simulink model "tricopter_simulation"  (Simulink 7.8)
settings: Solver=FixedStepDiscrete  StartTime=0.0  StopTime=10  FixedStep=dt_sim  RelTol=1e-3
InitFcn:
  | Init
values from neighbouring files (symbols this model uses):
  act_latency = 1*dt_sim    (= 0.005)    [Init.m]
  D = 1    [Init.m]
  dt_sim = 0.005    [Init.m]
  gvec = [0 0 9.81]'    [Init.m]
  J = diag([0.25*m*(D/2)^2 0.25*m*(D/2)^2 0.5*m*(D/2)^2])    [Init.m]
  k = 0.0000192    (= 1.92e-05)    [Init.m]
  L = 0.5    [Init.m]
  m = 1    [Init.m]
  max_rpm = 7000*pi/30    (= 733.038285838)    [Init.m]
  min_rpm = 0    [Init.m]
  rho = 1.26    [Init.m]
undefined symbols (not defined in the file or in its folder): DiscIntNeverNeededParam, waitfortreal
libraries: animation_lib x1, simulink x1
(part 2 of 2)

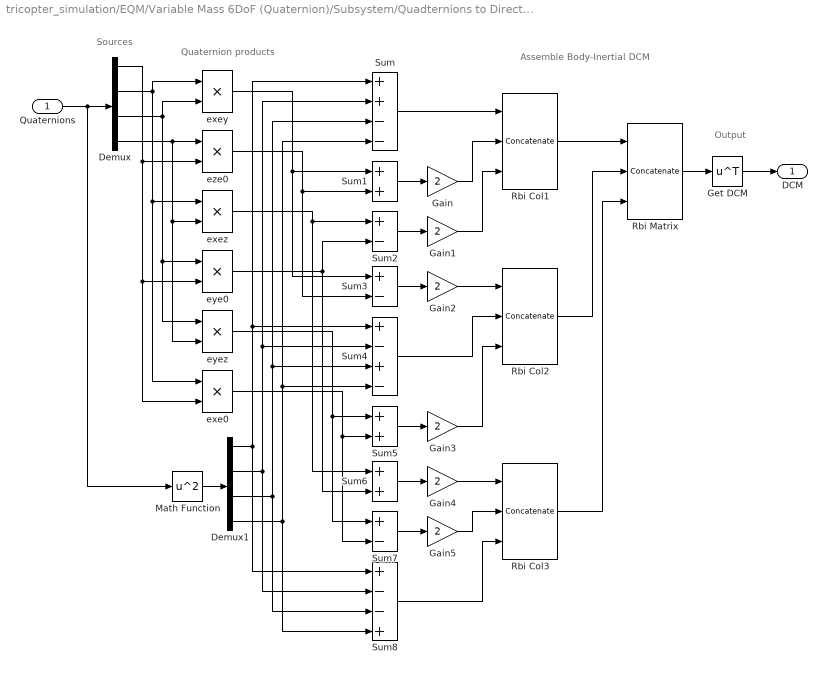
== system tricopter_simulation/EQM/Variable Mass 6DoF (Quaternion)/Subsystem/Quadternions to Direct Cosine Matrix ==
  note: Output
  note: Quaternion products
  note: Assemble Body-Inertial DCM
  note: Sources
  Quaternions : Inport  PortDimensions=[4 1]
  Demux : Demux
  Demux1 : Demux
  Gain{,1..5} (6 alike) : Gain  Gain=2  SaturateOnIntegerOverflow=on  OutDataTypeStr=Inherit: Same as input  ParamDataTypeStr=Inherit: Same as input
  Get DCM : Math  Operator=transpose  SaturateOnIntegerOverflow=on
  Math Function : Math  Operator=square  SaturateOnIntegerOverflow=on
  Rbi Matrix : Concatenate  NumInputs=3  Mode=Multidimensional array  ConcatenateDimension=2
  Rbi Col1 : Concatenate  NumInputs=3  Mode=Multidimensional array
  Rbi Col2 : Concatenate  NumInputs=3  Mode=Multidimensional array
  Rbi Col3 : Concatenate  NumInputs=3  Mode=Multidimensional array
  Sum : Sum  Inputs=++--  SaturateOnIntegerOverflow=on  InputSameDT=on  OutDataTypeStr=Inherit: Same as first input
  Sum1 : Sum  SaturateOnIntegerOverflow=on  InputSameDT=on  OutDataTypeStr=Inherit: Same as first input
  Sum2 : Sum  Inputs=+-  SaturateOnIntegerOverflow=on  InputSameDT=on  OutDataTypeStr=Inherit: Same as first input
  Sum3 : Sum  Inputs=+-  SaturateOnIntegerOverflow=on  InputSameDT=on  OutDataTypeStr=Inherit: Same as first input
  Sum4 : Sum  Inputs=+-+-  SaturateOnIntegerOverflow=on  InputSameDT=on  OutDataTypeStr=Inherit: Same as first input
  Sum5 : Sum  SaturateOnIntegerOverflow=on  InputSameDT=on  OutDataTypeStr=Inherit: Same as first input
  Sum6 : Sum  SaturateOnIntegerOverflow=on  InputSameDT=on  OutDataTypeStr=Inherit: Same as first input
  Sum7 : Sum  Inputs=+-  SaturateOnIntegerOverflow=on  InputSameDT=on  OutDataTypeStr=Inherit: Same as first input
  Sum8 : Sum  Inputs=+--+  SaturateOnIntegerOverflow=on  InputSameDT=on  OutDataTypeStr=Inherit: Same as first input
  exe0 : Product  SaturateOnIntegerOverflow=on  InputSameDT=on  OutDataTypeStr=Inherit: Same as first input
  exey : Product  SaturateOnIntegerOverflow=on  InputSameDT=on  OutDataTypeStr=Inherit: Same as first input
  exez : Product  SaturateOnIntegerOverflow=on  InputSameDT=on  OutDataTypeStr=Inherit: Same as first input
  eye0 : Product  SaturateOnIntegerOverflow=on  InputSameDT=on  OutDataTypeStr=Inherit: Same as first input
  eyez : Product  SaturateOnIntegerOverflow=on  InputSameDT=on  OutDataTypeStr=Inherit: Same as first input
  eze0 : Product  SaturateOnIntegerOverflow=on  InputSameDT=on  OutDataTypeStr=Inherit: Same as first input
  DCM : Outport
  wires:
  Get DCM/1 -> DCM/1
  Rbi Matrix/1 -> Get DCM/1
  Sum8/1 -> Rbi Col3/3
  Gain5/1 -> Rbi Col3/2
  Gain4/1 -> Rbi Col3/1
  Rbi Col3/1 -> Rbi Matrix/3
  Sum7/1 -> Gain5/1
  Sum6/1 -> Gain4/1
  Rbi Col2/1 -> Rbi Matrix/2
  Gain3/1 -> Rbi Col2/3
  Sum4/1 -> Rbi Col2/2
  Gain2/1 -> Rbi Col2/1
  Sum5/1 -> Gain3/1
  Sum3/1 -> Gain2/1
  Rbi Col1/1 -> Rbi Matrix/1
  Gain1/1 -> Rbi Col1/3
  Gain/1 -> Rbi Col1/2
  Sum/1 -> Rbi Col1/1
  Sum2/1 -> Gain1/1
  Sum1/1 -> Gain/1
  exe0/1 -> Sum5/2, Sum7/2
  eyez/1 -> Sum5/1, Sum7/1
  eye0/1 -> Sum2/2, Sum6/2
  exez/1 -> Sum2/1, Sum6/1
  eze0/1 -> Sum1/2, Sum3/2
  exey/1 -> Sum1/1, Sum3/1
  Math Function/1 -> Demux1/1
  Demux/4 -> eze0/1, exez/2, eyez/2
  Demux/3 -> exey/2, eye0/1, eyez/1
  Demux/2 -> exey/1, exez/1, exe0/1
  Demux/1 -> eze0/2, eye0/2, exe0/2
  Quaternions/1 -> Demux/1, Math Function/1
  Demux1/1 -> Sum/1, Sum4/1, Sum8/1
  Demux1/2 -> Sum/2, Sum4/2, Sum8/2
  Demux1/3 -> Sum/3, Sum4/3, Sum8/3
  Demux1/4 -> Sum/4, Sum4/4, Sum8/4

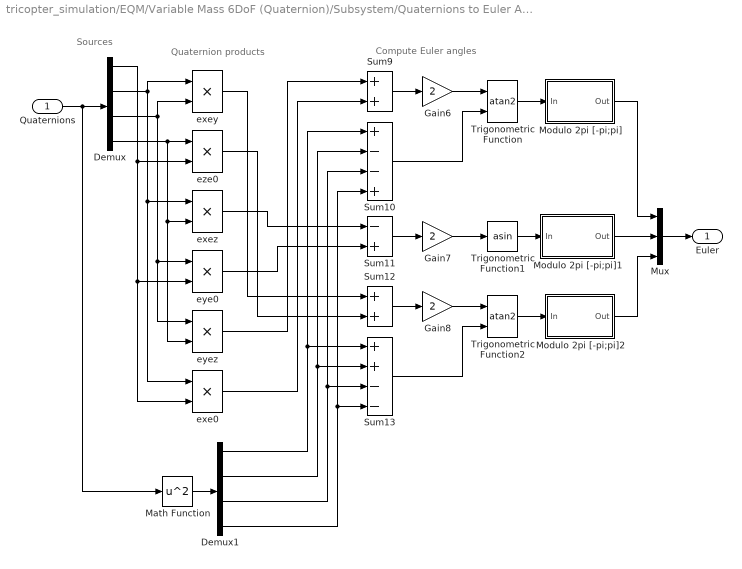
== system tricopter_simulation/EQM/Variable Mass 6DoF (Quaternion)/Subsystem/Quaternions to Euler Angles  ==
  note: Compute Euler angles
  note: Sources
  note: Quaternion products
  Quaternions : Inport  PortDimensions=[4 1]
  Demux : Demux
  Demux1 : Demux
  Gain6 : Gain  Gain=2  SaturateOnIntegerOverflow=on  OutDataTypeStr=Inherit: Same as input  ParamDataTypeStr=Inherit: Same as input
  Gain7 : Gain  Gain=2  SaturateOnIntegerOverflow=on  OutDataTypeStr=Inherit: Same as input  ParamDataTypeStr=Inherit: Same as input
  Gain8 : Gain  Gain=2  SaturateOnIntegerOverflow=on  OutDataTypeStr=Inherit: Same as input  ParamDataTypeStr=Inherit: Same as input
  Math Function : Math  Operator=square  SaturateOnIntegerOverflow=on
  Modulo 2pi [-pi;pi] : Subsystem
  Modulo 2pi [-pi;pi]1 : Subsystem
  Modulo 2pi [-pi;pi]2 : Subsystem
  Mux : Mux  Inputs=3
  Sum10 : Sum  Inputs=+--+  SaturateOnIntegerOverflow=on  InputSameDT=on  OutDataTypeStr=Inherit: Same as first input
  Sum11 : Sum  Inputs=-+  SaturateOnIntegerOverflow=on  InputSameDT=on  OutDataTypeStr=Inherit: Same as first input
  Sum12 : Sum  SaturateOnIntegerOverflow=on  InputSameDT=on  OutDataTypeStr=Inherit: Same as first input
  Sum13 : Sum  Inputs=++--  SaturateOnIntegerOverflow=on  InputSameDT=on  OutDataTypeStr=Inherit: Same as first input
  Sum9 : Sum  SaturateOnIntegerOverflow=on  InputSameDT=on  OutDataTypeStr=Inherit: Same as first input
  Trigonometric Function : Trigonometry  Operator=atan2
  Trigonometric Function1 : Trigonometry  Operator=asin
  Trigonometric Function2 : Trigonometry  Operator=atan2
  exe0 : Product  SaturateOnIntegerOverflow=on  InputSameDT=on  OutDataTypeStr=Inherit: Same as first input
  exey : Product  SaturateOnIntegerOverflow=on  InputSameDT=on  OutDataTypeStr=Inherit: Same as first input
  exez : Product  SaturateOnIntegerOverflow=on  InputSameDT=on  OutDataTypeStr=Inherit: Same as first input
  eye0 : Product  SaturateOnIntegerOverflow=on  InputSameDT=on  OutDataTypeStr=Inherit: Same as first input
  eyez : Product  SaturateOnIntegerOverflow=on  InputSameDT=on  OutDataTypeStr=Inherit: Same as first input
  eze0 : Product  SaturateOnIntegerOverflow=on  InputSameDT=on  OutDataTypeStr=Inherit: Same as first input
  Euler : Outport
  wires:
  Sum9/1 -> Gain6/1
  Gain6/1 -> Trigonometric Function/1
  Sum10/1 -> Trigonometric Function/2
  Sum11/1 -> Gain7/1
  Gain7/1 -> Trigonometric Function1/1
  Sum12/1 -> Gain8/1
  Gain8/1 -> Trigonometric Function2/1
  Sum13/1 -> Trigonometric Function2/2
  Trigonometric Function1/1 -> Modulo 2pi [-pi;pi]1/1(In)
  Trigonometric Function/1 -> Modulo 2pi [-pi;pi]/1(In)
  Trigonometric Function2/1 -> Modulo 2pi [-pi;pi]2/1(In)
  Quaternions/1 -> Demux/1, Math Function/1
  Demux/1 -> eze0/2, eye0/2, exe0/2
  Demux/2 -> exey/1, exez/1, exe0/1
  Demux/3 -> exey/2, eye0/1, eyez/1
  Demux/4 -> eze0/1, exez/2, eyez/2
  Demux1/1 -> Sum10/1, Sum13/1
  Demux1/2 -> Sum10/2, Sum13/2
  Demux1/3 -> Sum10/3, Sum13/3
  Demux1/4 -> Sum10/4, Sum13/4
  Math Function/1 -> Demux1/1
  exey/1 -> Sum12/1
  eze0/1 -> Sum12/2
  exez/1 -> Sum11/1
  eye0/1 -> Sum11/2
  eyez/1 -> Sum9/1
  exe0/1 -> Sum9/2
  Mux/1 -> Euler/1
  Modulo 2pi [-pi;pi]/1(Out) -> Mux/1
  Modulo 2pi [-pi;pi]1/1(Out) -> Mux/2
  Modulo 2pi [-pi;pi]2/1(Out) -> Mux/3

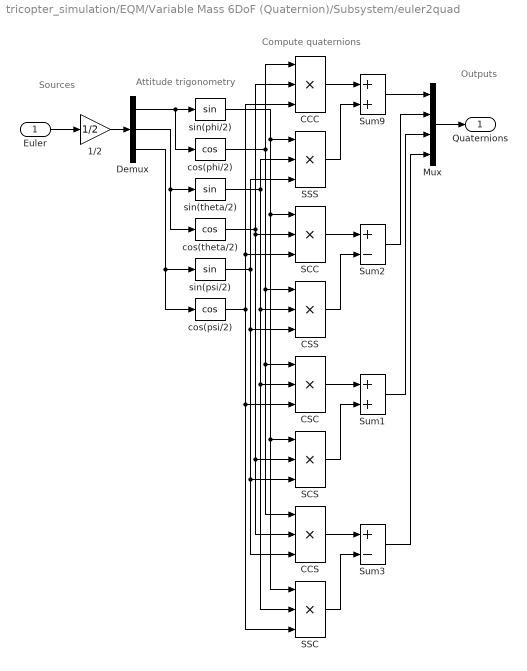
== system tricopter_simulation/EQM/Variable Mass 6DoF (Quaternion)/Subsystem/euler2quad ==
  note: Sources
  note: Attitude trigonometry
  note: Compute quaternions
  note: Outputs
  Euler : Inport  PortDimensions=[3 1]
  1/2 : Gain  Gain=1/2  SaturateOnIntegerOverflow=on  OutDataTypeStr=Inherit: Same as input  ParamDataTypeStr=Inherit: Same as input
  CCC : Product  Inputs=3  SaturateOnIntegerOverflow=on  InputSameDT=on  OutDataTypeStr=Inherit: Same as first input
  CCS : Product  Inputs=3  SaturateOnIntegerOverflow=on  InputSameDT=on  OutDataTypeStr=Inherit: Same as first input
  CSC : Product  Inputs=3  SaturateOnIntegerOverflow=on  InputSameDT=on  OutDataTypeStr=Inherit: Same as first input
  CSS : Product  Inputs=3  SaturateOnIntegerOverflow=on  InputSameDT=on  OutDataTypeStr=Inherit: Same as first input
  Demux : Demux  Outputs=3
  Mux : Mux
  SCC : Product  Inputs=3  SaturateOnIntegerOverflow=on  InputSameDT=on  OutDataTypeStr=Inherit: Same as first input
  SCS : Product  Inputs=3  SaturateOnIntegerOverflow=on  InputSameDT=on  OutDataTypeStr=Inherit: Same as first input
  SSC : Product  Inputs=3  SaturateOnIntegerOverflow=on  InputSameDT=on  OutDataTypeStr=Inherit: Same as first input
  SSS : Product  Inputs=3  SaturateOnIntegerOverflow=on  InputSameDT=on  OutDataTypeStr=Inherit: Same as first input
  Sum1 : Sum  SaturateOnIntegerOverflow=on  InputSameDT=on  OutDataTypeStr=Inherit: Same as first input
  Sum2 : Sum  Inputs=+-  SaturateOnIntegerOverflow=on  InputSameDT=on  OutDataTypeStr=Inherit: Same as first input
  Sum3 : Sum  Inputs=+-  SaturateOnIntegerOverflow=on  InputSameDT=on  OutDataTypeStr=Inherit: Same as first input
  Sum9 : Sum  SaturateOnIntegerOverflow=on  InputSameDT=on  OutDataTypeStr=Inherit: Same as first input
  cos(phi/2) : Trigonometry  Operator=cos
  cos(psi/2) : Trigonometry  Operator=cos
  cos(theta/2) : Trigonometry  Operator=cos
  sin(phi/2) : Trigonometry
  sin(psi/2) : Trigonometry
  sin(theta/2) : Trigonometry
  Quaternions : Outport
  wires:
  Mux/1 -> Quaternions/1
  Euler/1 -> 1/2/1
  1/2/1 -> Demux/1
  Demux/1 -> sin(phi/2)/1, cos(phi/2)/1
  Demux/2 -> cos(theta/2)/1, sin(theta/2)/1
  Demux/3 -> cos(psi/2)/1, sin(psi/2)/1
  cos(psi/2)/1 -> CCC/3, SCC/3, SSC/3, CSC/3
  sin(psi/2)/1 -> SSS/3, CSS/3, CCS/3, SCS/3
  cos(theta/2)/1 -> SCC/2, CCS/2, SCS/2, CCC/2
  sin(theta/2)/1 -> SSS/2, CSS/2, SSC/2, CSC/2
  cos(phi/2)/1 -> CSS/1, CCS/1, CSC/1, CCC/1
  sin(phi/2)/1 -> SCC/1, SSC/1, SCS/1, SSS/1
  CCC/1 -> Sum9/1
  SSS/1 -> Sum9/2
  CSC/1 -> Sum1/1
  SCS/1 -> Sum1/2
  SCC/1 -> Sum2/1
  CSS/1 -> Sum2/2
  CCS/1 -> Sum3/1
  SSC/1 -> Sum3/2
  Sum9/1 -> Mux/1
  Sum2/1 -> Mux/2
  Sum1/1 -> Mux/3
  Sum3/1 -> Mux/4

== system tricopter_simulation/EQM/Variable Mass 6DoF (Quaternion)/Subsystem/Body Rates Integration/Rate Integration ==
  p q r : Inport
  q0 q1 q2 q3 : Inport  Port=2
  Gain : Gain  Gain=dt_sim
  Gain2 : Gain  Gain=0.5
  Magnitude 3d : Subsystem
      mask Type: Magnitude Square
      mask Description:
      | Magnitude of a 3-dimensional vector.
      | Input: 3-d vector (x,y,z).
      | Output: magn = sqrt(x^2 + y^2 + z^2).
      mask Help: Unmask block for more help.
      mask Display: disp('sqrt(x^2+y^2+z^2)')
  Mux : Mux  Inputs=2
  Normalization : Subsystem
      mask Type: Vector normalization
      mask Description: Normalize a vector, e = v/|v|.
      mask Help:
      | The block normalizes the input vector.
      | <P><B>Input:</B> the nx1 vector;</P>
      | <P><B>Output:</B> the nx1 unit vector.</P>
  Product : Product  RndMeth=Zero
  Quaternion Product : Subsystem
  Trigonometric Function : Trigonometry
  Trigonometric Function1 : Trigonometry  Operator=cos  OutputSignalType=real
  q_prod : Outport  InitialOutput=0
  wires:
  q0 q1 q2 q3/1 -> Quaternion Product/1(q_x)
  Quaternion Product/1(q) -> q_prod/1
  p q r/1 -> Gain/1, Normalization/1(VecIn)
  Magnitude 3d/1(out) -> Gain2/1
  Gain2/1 -> Trigonometric Function/1, Trigonometric Function1/1  "delta/2"
  Trigonometric Function1/1 -> Mux/1
  Trigonometric Function/1 -> Product/1
  Normalization/1(VecOut) -> Product/2  "vector n"
  Product/1 -> Mux/2
  Gain/1 -> Magnitude 3d/1(in)
  Mux/1 -> Quaternion Product/2(q_y)

== system tricopter_simulation/EQM/Variable Mass 6DoF (Quaternion)/Subsystem/Quaternions to Euler Angles /Modulo 2pi [-pi;pi] ==
  In : Inport
  " " : Constant  Value=2*pi
  "  " : Constant  Value=pi
  "     " : Constant  Value=pi
  Math Function : Math  Operator=mod  SaturateOnIntegerOverflow=on
  Sum2 : Sum  Inputs=|++  SaturateOnIntegerOverflow=on  InputSameDT=on  OutDataTypeStr=Inherit: Same as first input
  Sum3 : Sum  Inputs=|+-  SaturateOnIntegerOverflow=on  InputSameDT=on  OutDataTypeStr=Inherit: Same as first input
  Out : Outport
  wires:
  In/1 -> Sum2/1
  Sum3/1 -> Out/1
  "     "/1 -> Sum2/2
  "  "/1 -> Sum3/2
  Sum2/1 -> Math Function/1
  Math Function/1 -> Sum3/1
  " "/1 -> Math Function/2

== system tricopter_simulation/EQM/Variable Mass 6DoF (Quaternion)/Subsystem/Quaternions to Euler Angles /Modulo 2pi [-pi;pi]1 ==
  In : Inport
  " " : Constant  Value=2*pi
  "  " : Constant  Value=pi
  "     " : Constant  Value=pi
  Math Function : Math  Operator=mod  SaturateOnIntegerOverflow=on
  Sum2 : Sum  Inputs=|++  SaturateOnIntegerOverflow=on  InputSameDT=on  OutDataTypeStr=Inherit: Same as first input
  Sum3 : Sum  Inputs=|+-  SaturateOnIntegerOverflow=on  InputSameDT=on  OutDataTypeStr=Inherit: Same as first input
  Out : Outport
  wires:
  " "/1 -> Math Function/2
  Math Function/1 -> Sum3/1
  Sum2/1 -> Math Function/1
  "  "/1 -> Sum3/2
  "     "/1 -> Sum2/2
  Sum3/1 -> Out/1
  In/1 -> Sum2/1

== system tricopter_simulation/EQM/Variable Mass 6DoF (Quaternion)/Subsystem/Quaternions to Euler Angles /Modulo 2pi [-pi;pi]2 ==
  In : Inport
  " " : Constant  Value=2*pi
  "  " : Constant  Value=pi
  "     " : Constant  Value=pi
  Math Function : Math  Operator=mod  SaturateOnIntegerOverflow=on
  Sum2 : Sum  Inputs=|++  SaturateOnIntegerOverflow=on  InputSameDT=on  OutDataTypeStr=Inherit: Same as first input
  Sum3 : Sum  Inputs=|+-  SaturateOnIntegerOverflow=on  InputSameDT=on  OutDataTypeStr=Inherit: Same as first input
  Out : Outport
  wires:
  In/1 -> Sum2/1
  Sum3/1 -> Out/1
  "     "/1 -> Sum2/2
  "  "/1 -> Sum3/2
  Sum2/1 -> Math Function/1
  Math Function/1 -> Sum3/1
  " "/1 -> Math Function/2

== system tricopter_simulation/EQM/Variable Mass 6DoF (Quaternion)/Subsystem/Body Rates Integration/Rate Integration/Magnitude 3d ==
  note: magnitude for 3-d vector
  in : Inport
  Signal Specification : SignalSpecification  Dimensions=3
  magnitude square : Fcn  Expr=sqrt(u[1]*u[1]+u[2]*u[2]+u[3]*u[3])
  out : Outport
  wires:
  Signal Specification/1 -> magnitude square/1
  in/1 -> Signal Specification/1
  magnitude square/1 -> out/1

== system tricopter_simulation/EQM/Variable Mass 6DoF (Quaternion)/Subsystem/Body Rates Integration/Rate Integration/Normalization ==
  VecIn : Inport
  Switch : Switch  Criteria=u2 > Threshold  Threshold=0.0001  InputSameDT=on
  Vector norm : Subsystem
      mask Type: Vector norm-2
      mask Description: Compute the 2-norm (magnitude) of a vector, |v| = sqrt(v'v)
  e/|e| : Product  Inputs=*/  SaturateOnIntegerOverflow=on  InputSameDT=on  OutDataTypeStr=Inherit: Same as first input
  VecOut : Outport
  wires:
  Vector norm/1(Mag) -> e/|e|/2, Switch/2
  e/|e|/1 -> Switch/1
  VecIn/1 -> e/|e|/1, Vector norm/1(Vec), Switch/3
  Switch/1 -> VecOut/1

== system tricopter_simulation/EQM/Variable Mass 6DoF (Quaternion)/Subsystem/Body Rates Integration/Rate Integration/Quaternion Product ==
  q_x : Inport
  q_y : Inport  Port=2
  Pathfixed = 2 : Mux  Inputs=2
  Pathfixed = 4 : Mux
  Reshape : Reshape
  Reshape1 : Reshape
  q_0 : Fcn  Expr=u[1] * u[5] - u[2] * u[6] - u[3] * u[7] - u[4] * u[8]
  q_1 : Fcn  Expr=u[1] * u[6] + u[2] * u[5] + u[3] * u[8] - u[4] * u[7]
  q_2 : Fcn  Expr=u[1] * u[7] - u[2] * u[8] + u[3] * u[5] + u[4] * u[6]
  q_3 : Fcn  Expr=u[1] * u[8] + u[2] * u[7] - u[3] * u[6] + u[4] * u[5]
  q : Outport
  wires:
  Reshape1/1 -> Pathfixed = 2/2
  Reshape/1 -> Pathfixed = 2/1
  Pathfixed = 2/1 -> q_0/1, q_1/1, q_2/1, q_3/1
  q_0/1 -> Pathfixed = 4/1
  q_1/1 -> Pathfixed = 4/2
  q_2/1 -> Pathfixed = 4/3
  q_3/1 -> Pathfixed = 4/4
  q_x/1 -> Reshape/1
  Pathfixed = 4/1 -> q/1
  q_y/1 -> Reshape1/1

== system tricopter_simulation/EQM/Variable Mass 6DoF (Quaternion)/Subsystem/Body Rates Integration/Rate Integration/Normalization/Vector norm ==
  Vec : Inport
  Dot Product : DotProduct  InputSameDT=on  OutDataTypeStr=Inherit: Inherit via internal rule
  Sqrt : Sqrt  OutputSignalType=real  SaturateOnIntegerOverflow=on
  Mag : Outport
  wires:
  Sqrt/1 -> Mag/1
  Dot Product/1 -> Sqrt/1
  Vec/1 -> Dot Product/2, Dot Product/1

== matlab function KK-Controller/MATLAB Function ==
  data: RxChannelLat input double; RxChannelLon input double; RxChannelCol input double; RxChannelPed input double; MotorOut1 output double; p input double; q input double; r input double; KProll input double; KPpitch input double; KPyaw input double; integral_in input double size=3; last_error_in input double size=3; MotorOut2 output double; MotorOut3 output double; MotorOut4 output double; integral_out output double; last_error_out output double
function [MotorOut1, MotorOut2, MotorOut3, MotorOut4, integral_out, last_error_out] = KKcontroller(RxChannelLat, RxChannelLon, RxChannelCol,RxChannelPed ,  p, q, r, KProll, KPpitch, KPyaw, integral_in, last_error_in)
%https://github.com/sim-/kk/blob/master/kk.c

ROLL = 1;   % roll index definition
PITCH = 2;  % pitch index definition
YAW = 3;    % yaw index definition

emax = 1023;


integral = integral_in;
last_error = last_error_in;

RxInRoll = RxChannelLat - 1500;
RxInPitch = RxChannelLon - 1500;
RxInCollective = RxChannelCol - 1100;
RxInYaw = RxChannelPed - 1500;

%-------------------------------------------------------
%--- Start mixing by setting collective to motor outputs
%-------------------------------------------------------
RxInCollective = (RxInCollective * 10) /8;	% 0-800 -> 0-1000
MotorOut1 = RxInCollective;
MotorOut2 = RxInCollective;
MotorOut3 = RxInCollective;
MotorOut4 = 500;

%-------------------------------------------------------
% Roll control loop
%-------------------------------------------------------
error = KProll*(RxInRoll - p);
if (error > emax)
    error = emax;
elseif (error < -emax)
        error = -emax;
end
    
integral(ROLL) = integral(ROLL) + error;

imax = RxInCollective;
if (imax < 0)
    imax = 0;
end

imax = imax/10;	% 1000 -> 200
if (integral(ROLL) > imax)
    integral(ROLL) = imax;
elseif (integral(ROLL) < -imax)
        integral(ROLL) = -imax;
end

derivative = error - last_error(ROLL);
last_error(ROLL) = error;
RxInRoll = RxInRoll + error;% + (integral(ROLL) / 4) + (derivative / 4);

% [Tricopter]
RxInRoll = RxInRoll * 0.875; 
% (RxInRoll * 7) >> 3 = RxInRoll*0.875 Approximation of sin(60)=(.875 versus .86602540) without div
MotorOut1 = MotorOut1 + RxInRoll;
MotorOut2 = MotorOut2 - RxInRoll;

%-------------------------------------------------------
% Pitch control loop
%-------------------------------------------------------
error = KPpitch*(RxInPitch  - q);
if (error > emax)
    error = emax;
elseif (error < -emax)
        error = -emax;
end
    
integral(PITCH) = integral(PITCH) + error;

if (integral(PITCH) > imax)
    integral(PITCH) = imax;
elseif (integral(PITCH) < -imax)
        integral(PITCH) = -imax;
end

derivative = error - last_error(PITCH);
last_error(PITCH) = error;
RxInPitch = RxInPitch + error;% + (integral(PITCH) / 4) + (derivative / 4);

% [Tricopter]
MotorOut3 = MotorOut3 - RxInPitch;
RxInPitch = RxInPitch /2;   % cosine of 60
MotorOut1 = MotorOut1 + RxInPitch;
MotorOut2 = MotorOut2 + RxInPitch;

%-------------------------------------------------------
% Yaw control loop
%-------------------------------------------------------
error = KPyaw*(RxInYaw  - r);
if (error > emax)
    error = emax;
elseif (error < -emax)
        error = -emax;
end
    
integral(YAW) = integral(YAW) + error;

if (integral(YAW) > imax)
    integral(YAW) = imax;
elseif (integral(YAW) < -imax)
        integral(YAW) = -imax;
end

derivative = error - last_error(YAW);
last_error(YAW) = error;
RxInYaw = RxInYaw + error;% + (integral(YAW) / 4) + (derivative / 4);

% [Tricopter]
MotorOut4 = MotorOut4 + RxInYaw;


% [Tricopter]
% Rather than clipping the motor outputs and causing instability
% at throttle saturation, we pull down the throttle of the other
% motors. This gives priority to stabilization without a fixed
% collective limit.

imax = MotorOut1;
if (MotorOut2 > imax)
    imax = MotorOut2;
end
if (MotorOut3 > imax)
    imax = MotorOut3;
end
imax = imax - 1000;
if (imax > 0) 
    MotorOut1 = MotorOut1 - imax;
    MotorOut2 = MotorOut2 - imax;
    MotorOut3 = MotorOut3 - imax;
end

%--- Limit the lowest value to avoid stopping of motor if motor value is under-saturated ---
imax = 114;             % this is the motor idle level
if (MotorOut1 < imax)
    MotorOut1 = imax;	
end
if (MotorOut2 < imax)
    MotorOut2 = imax;
end

%#if defined(TRI_COPTER) || defined(QUAD_COPTER) || defined(QUAD_X_COPTER) || defined(Y4_COPTER)
if (MotorOut3 < imax)
    MotorOut3 = imax;
end

% Bound pulse length to 1ms <= pulse <= 2ms
MotorOut1 = MotorOut1 +1000;
MotorOut2 = MotorOut2 +1000;
MotorOut3 = MotorOut3 +1000;
MotorOut4 = MotorOut4 +1000;

integral_out = integral;
last_error_out = last_error;
